simulink model "noise_model_simulink"  (R2019a)
settings: Solver=VariableStepAuto  StartTime=0.0  StopTime=60  RelTol=1e-3
libraries: dspsrcs4 x1
settings Model: Creator=Carolina  LastModifiedBy=Carolina

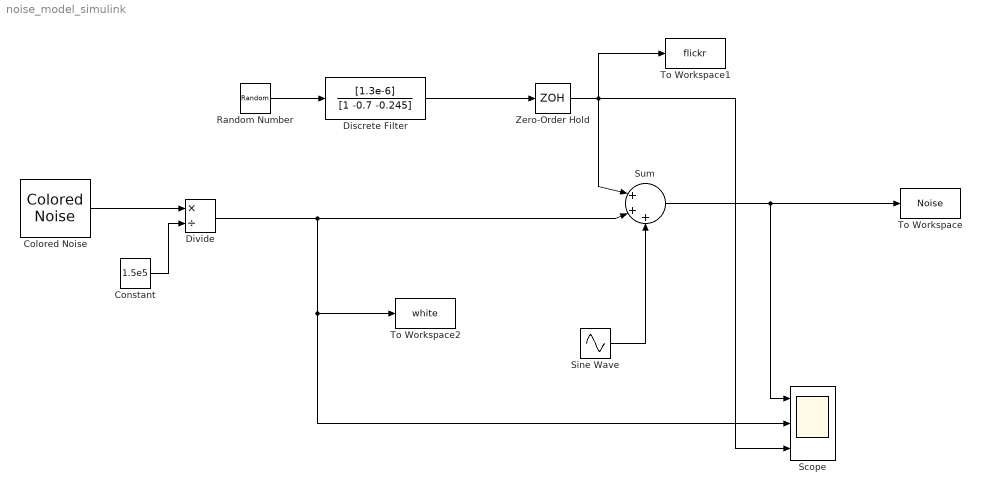
== system noise_model_simulink ==
  Colored Noise : dspsrcs4/Colored Noise  Color=white  InverseFrequencyPower=1  NumChannels=1  OutputDataType=double  SamplesPerFrame=1  SampleTime=1/24414  RandomStream=mt19937ar with seed  Seed=67  SimulateUsing=Interpreted execution
      settings: SourceProductName=DSP System Toolbox  SourceProductBaseCode=DS
  Constant : Constant  Value=1.5e5
  Discrete Filter : DiscreteFilter  Numerator=[1.3e-6]  Denominator=[1 -0.7 -0.245]
  Divide : Product  Inputs=*/
  Random Number : RandomNumber  SampleTime=1/24414
  Scope : Scope  NumInputPorts=3
  Sine Wave : Sin  Amplitude=0.6e-6  Frequency=314.16  SampleTime=1/24414
  Sum : Sum  Inputs=|+++
  To Workspace : ToWorkspace  VariableName=Noise  SaveFormat=Structure With Time  SampleTime=-1
  To Workspace1 : ToWorkspace  VariableName=flickr  SaveFormat=Structure With Time  SampleTime=-1
  To Workspace2 : ToWorkspace  VariableName=white  SaveFormat=Structure With Time  SampleTime=-1
  Zero-Order Hold : ZeroOrderHold  SampleTime=-1
  wires:
  Discrete Filter/1 -> Zero-Order Hold/1
  Sine Wave/1 -> Sum/3
  Sum/1 -> Scope/1, To Workspace/1
  Random Number/1 -> Discrete Filter/1
  Colored Noise/1 -> Divide/1
  Divide/1 -> To Workspace2/1, Scope/2, Sum/2
  Constant/1 -> Divide/2
  Zero-Order Hold/1 -> Sum/1, To Workspace1/1, Scope/3
